simulink model "simpleHelicopter"  (R2024a)
settings: Solver=FixedStepAuto  StartTime=0.0  StopTime=500  FixedStep=fixedStepSize  RelTol=1e-3
model workspace: external: MATLAB File .\turboShaftEngine\Scripts\Initialization\initialization.m (data not in the file)
libraries: fl_lib x4, nesl_utility x3, simulink x2, aerolibatmos2 x1, SignalEditorBlockLib x1
settings Model: DataDictionary=initialization.sldd  EnableAccessToBaseWorkspace=off  Creator=imyrsini  LastModifiedBy=imyrsini
settings OptimizationCC: ZeroExternalMemoryAtStartup=off  ZeroInternalMemoryAtStartup=off
settings RTWCC: TargetLang=C++  GPUComputeCapability=3.5
settings GRTTargetCC: TargetLangStandard=C++11 (ISO)  CodeInterfacePackaging=C++ class
settings SimscapeCC: SimscapeLogSimulationStatistics=on  SimscapeLogToSDI=on  SimscapeLogLimitData=off

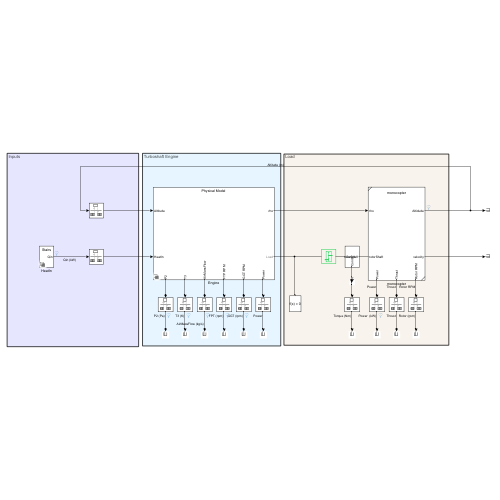
[thumbnail: Simulink's stored preview of the top-level diagram]
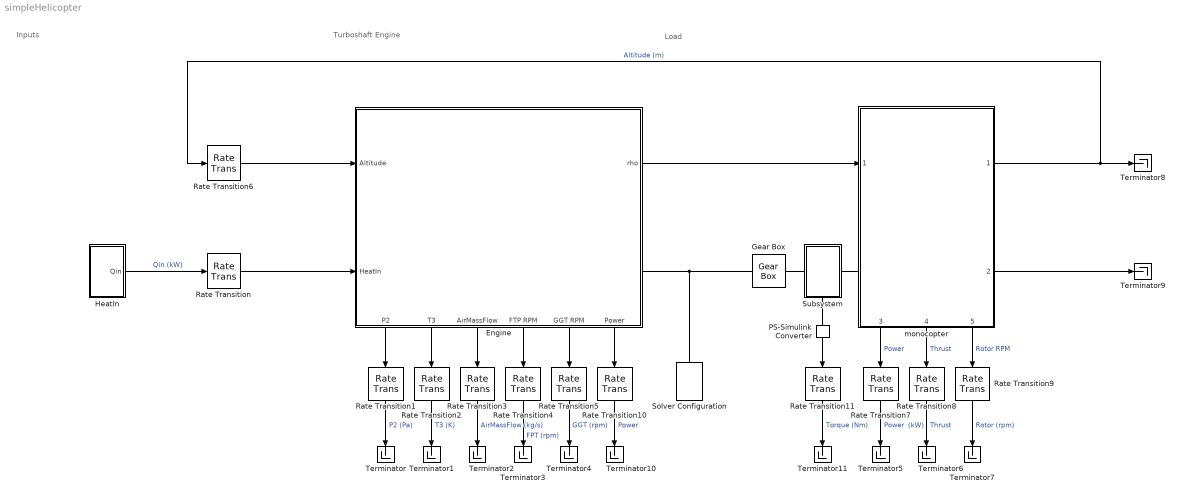
== system simpleHelicopter ==
  note: Load
  note: Turboshaft Engine
  note: Inputs
  Engine : Subsystem  Variant=on  VariantControlMode=label  VariantControl=Subsystem  LabelModeActiveChoice=PhysMod
      settings: PortSchema="{\"entries\":[{\"content\":{\"sides\":[{\"content\":{\"connectorIds\":[\"In1\",\"In2\"]},\"type\":\"ConnectorPlacement.EquallySpacedRectSide\",\"uuid\":\"4b97c1b6-1ef0-4aa6-ad92-ebabb24ed618\"},{\"content\":{\"connectorIds\":[\"Out1\",\"RConn1\"],\"side\":\"RIGHT\"},\"type\":\"ConnectorPlacement.EquallySpacedRectSide\",\"uuid\":\"48732025-ee88-4ad0-bb4a-c439796f910a\"},{\"content\":{\"side\":\"TOP\"},\"type\":\"ConnectorPlacement.EquallySpacedRectSide\",\"uuid\":\"e2101b7b-5c5b-49a6-a3d3-6276ba2fcf7e\"},{\"content\":{\"connectorIds\":[\"Out2\",\"Out3\",\"Out4\",\"Out5\",\"Out6\",\"Out7\"],\"side\":\"BOTTOM\"},\"type\":\"ConnectorPlacement.EquallySpacedRectSide\",\"uuid\":\"1d0ac715-4d03-40bf-a736-541001f37f0a\"}]},\"type\":\"ConnectorPlacement.EquallySpacedConnector\",\"uuid\":\"cc865452-eabe-4ee6-a5dd-432e5e4e603b\"}],\"packageUris\":[\"http://schema.mathworks.com/mf0/Connector/R2020b\"],\"version\":\"1.0\"}"
  Gear Box : fl_lib/Mechanical/Mechanisms/Gear Box  ratio=shaftFTP.GearRatio  t_in_specify=off  t_in_priority=None  t_in=0 N*m  t_in_nominal_specify=off  t_in_nominal_value=1  t_in_nominal_unit=N*m  t_out_specify=off  t_out_priority=None  t_out=0 N*m  t_out_nominal_specify=off  t_out_nominal_value=1  t_out_nominal_unit=N*m
  HeatIn : Subsystem  Variant=on  VariantControlMode=label  VariantControl=Choice  LabelModeActiveChoice=Stairs
  PS-Simulink Converter : nesl_utility/PS-Simulink Converter  PhysicalDomain=network_engine_domain  SubClassName=ps_output  LeftPortType=input  RightPortType=output  PseudoPeriodic=off  Frequencies=[]  VectorFormat=inherit  Unit=inherit  AffineConversion=off
  Rate Transition{,1..11} (12 alike) : RateTransition  Integrity=off
  Solver Configuration : nesl_utility/Solver Configuration  PhysicalDomain=network_engine_domain  SubClassName=solver  LeftPortType=input  RightPortType=generic  Tones=[]  Harmonics=[]  SimulateNoise=off  Profile=off  UseLocalSampling=off  EnableSwitchedLinearOptims=on  FrequencyDomain=off  UseCCode=off  RelTol=0.001  AbsTol=0.001  MinStep=1e-09  ToWorkspace=off  RevertToSquareIcSolve=off  NumHomotopyIterations=100  PhasorMode=off  PhasorModeNumHarmonics=1  ConsistencySolver=NEWTON_XTOL_AFTER_FTOL  IndexReductionMethod=DerivativeReplacement  DoDC=on  ResidualTolerance=1e-09  ConsistencyTolSource=GLOBAL  ConsistencyAbsTol=0.001  ConsistencyRelTol=0.001  ConsistencyTolFactor=0.001  UseLocalSolver=off  LocalSolverChoice=NE_BACKWARD_EULER_ADVANCER  ResolveIndetEquations=on  FunctionEvalNumThread=1  LocalSolverSampleTime=0.001  DoFixedCost=off  MaxNonlinIter=3  MaxModeIter=2  ComputeImpulses=off  ImpulseIterations=2  LinearAlgebra=auto  LinearAlgebraNumThread=0  EquationFormulation=NE_TIME_EF  DelaysMemoryBudget=1024  AutomaticFiltering=on  FilteringTimeConstant=0.001  PartitionStorageMethod=AS_NEEDED  PartitionMemoryBudget=1024  PartitionMethod=ROBUST  MultibodyUseLocalSolver=off  MultibodyLocalSolverChoice=ODE1  MultibodyLocalSolverSampleTime=0.001
  Subsystem : Subsystem
      settings: PortSchema="{\"entries\":[{\"content\":{\"sides\":[{\"content\":{\"connectorIds\":[\"LConn1\"]},\"type\":\"ConnectorPlacement.EquallySpacedRectSide\",\"uuid\":\"cd933ecd-5fe2-4a61-aaa8-d3fcacb54062\"},{\"content\":{\"connectorIds\":[\"RConn1\"],\"side\":\"RIGHT\"},\"type\":\"ConnectorPlacement.EquallySpacedRectSide\",\"uuid\":\"e8204415-45e5-46c1-88c3-e1f0a7c4e852\"},{\"content\":{\"side\":\"TOP\"},\"type\":\"ConnectorPlacement.EquallySpacedRectSide\",\"uuid\":\"484e5189-0a43-4f33-96ac-bd4f306fcf4f\"},{\"content\":{\"connectorIds\":[\"RConn2\"],\"side\":\"BOTTOM\"},\"type\":\"ConnectorPlacement.EquallySpacedRectSide\",\"uuid\":\"524c6b30-eaeb-4c5f-81b0-1e7f5997b042\"}]},\"type\":\"ConnectorPlacement.EquallySpacedConnector\",\"uuid\":\"7bdab1e5-ac38-4f53-a4df-032da561ec46\"}],\"packageUris\":[\"http://schema.mathworks.com/mf0/Connector/R2020b\"],\"version\":\"1.0\"}"
  Terminator{,1..11} (12 alike) : Terminator
  monocopter : Subsystem  ReferencedSubsystem=monocopter
      settings: PortSchema="{\"entries\":[{\"content\":{\"sides\":[{\"content\":{\"connectorIds\":[\"In1\",\"LConn1\"]},\"type\":\"ConnectorPlacement.EquallySpacedRectSide\",\"uuid\":\"2ecbf831-8a46-4c85-bf63-980a752dd5b1\"},{\"content\":{\"connectorIds\":[\"Out1\",\"Out2\"],\"side\":\"RIGHT\"},\"type\":\"ConnectorPlacement.EquallySpacedRectSide\",\"uuid\":\"e1b9456e-2a06-4a0b-bd2d-ca850f525143\"},{\"content\":{\"side\":\"TOP\"},\"type\":\"ConnectorPlacement.EquallySpacedRectSide\",\"uuid\":\"495d5151-b094-4c59-ad95-48151a95ddaf\"},{\"content\":{\"connectorIds\":[\"Out3\",\"Out4\",\"Out5\"],\"side\":\"BOTTOM\"},\"type\":\"ConnectorPlacement.EquallySpacedRectSide\",\"uuid\":\"d711d358-7c2d-4243-addb-9f7f6c9821dd\"}]},\"type\":\"ConnectorPlacement.EquallySpacedConnector\",\"uuid\":\"3949e89b-de6d-4024-bd06-1eddfa87edaa\"}],\"packageUris\":[\"http://schema.mathworks.com/mf0/Connector/R2020b\"],\"version\":\"1.0\"}"
  wires:
  HeatIn/1(Qin) -> Rate Transition/1  "Qin (kW)"
  monocopter/2 -> Terminator9/1
  monocopter/3 -> Rate Transition7/1  "Power"
  monocopter/4 -> Rate Transition8/1  "Thrust"
  monocopter/5 -> Rate Transition9/1  "Rotor RPM"
  monocopter/1 -> Terminator8/1, Rate Transition6/1  "Altitude (m)"
  Rate Transition7/1 -> Terminator5/1  "Power  (kW)"
  Rate Transition8/1 -> Terminator6/1  "Thrust"
  Rate Transition9/1 -> Terminator7/1  "Rotor (rpm)"
  Rate Transition6/1 -> Engine/1(Altitude)
  Rate Transition/1 -> Engine/2(HeatIn)
  Engine/1(rho) -> monocopter/1
  Engine/2(P2) -> Rate Transition1/1
  Engine/3(T3) -> Rate Transition2/1
  Engine/4(AirMassFlow) -> Rate Transition3/1
  Engine/5(FTP RPM) -> Rate Transition4/1
  Engine/6(GGT RPM) -> Rate Transition5/1
  Engine/7(Power) -> Rate Transition10/1
  Rate Transition1/1 -> Terminator/1  "P2 (Pa)"
  Rate Transition2/1 -> Terminator1/1  "T3 (K)"
  Rate Transition3/1 -> Terminator2/1  "AirMassFlow (kg/s)"
  Rate Transition4/1 -> Terminator3/1  "FPT (rpm)"
  Rate Transition5/1 -> Terminator4/1  "GGT (rpm)"
  Rate Transition10/1 -> Terminator10/1  "Power"
  PS-Simulink Converter/1 -> Rate Transition11/1
  Rate Transition11/1 -> Terminator11/1  "Torque (Nm)"
  connections:
  Solver Configuration/RConn1 -- Engine/RConn1 -- Gear Box/LConn1
  Subsystem/RConn1 -- Gear Box/RConn1
  Subsystem/LConn1 -- monocopter/LConn1
  Subsystem/RConn2 -- PS-Simulink Converter/LConn1

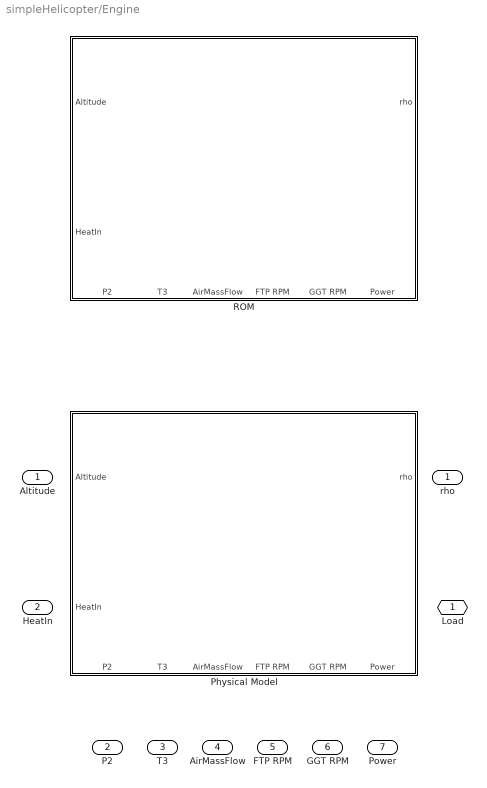
== system simpleHelicopter/Engine ==
  Altitude : Inport
  HeatIn : Inport  Port=2
  Physical Model : Subsystem  VariantControl=PhysMod
      settings: PortSchema="{\"entries\":[{\"content\":{\"sides\":[{\"content\":{\"connectorIds\":[\"In1\",\"In2\"]},\"type\":\"ConnectorPlacement.EquallySpacedRectSide\",\"uuid\":\"4b97c1b6-1ef0-4aa6-ad92-ebabb24ed618\"},{\"content\":{\"connectorIds\":[\"Out1\",\"RConn1\"],\"side\":\"RIGHT\"},\"type\":\"ConnectorPlacement.EquallySpacedRectSide\",\"uuid\":\"48732025-ee88-4ad0-bb4a-c439796f910a\"},{\"content\":{\"side\":\"TOP\"},\"type\":\"ConnectorPlacement.EquallySpacedRectSide\",\"uuid\":\"e2101b7b-5c5b-49a6-a3d3-6276ba2fcf7e\"},{\"content\":{\"connectorIds\":[\"Out2\",\"Out3\",\"Out4\",\"Out5\",\"Out6\",\"Out7\"],\"side\":\"BOTTOM\"},\"type\":\"ConnectorPlacement.EquallySpacedRectSide\",\"uuid\":\"1d0ac715-4d03-40bf-a736-541001f37f0a\"}]},\"type\":\"ConnectorPlacement.EquallySpacedConnector\",\"uuid\":\"cc865452-eabe-4ee6-a5dd-432e5e4e603b\"}],\"packageUris\":[\"http://schema.mathworks.com/mf0/Connector/R2020b\"],\"version\":\"1.0\"}"
  ROM : Subsystem  VariantControl=ROM
      settings: PortSchema="{\"entries\":[{\"content\":{\"sides\":[{\"content\":{\"connectorIds\":[\"In1\",\"In2\"]},\"type\":\"ConnectorPlacement.EquallySpacedRectSide\",\"uuid\":\"4b97c1b6-1ef0-4aa6-ad92-ebabb24ed618\"},{\"content\":{\"connectorIds\":[\"Out1\",\"RConn1\"],\"side\":\"RIGHT\"},\"type\":\"ConnectorPlacement.EquallySpacedRectSide\",\"uuid\":\"48732025-ee88-4ad0-bb4a-c439796f910a\"},{\"content\":{\"side\":\"TOP\"},\"type\":\"ConnectorPlacement.EquallySpacedRectSide\",\"uuid\":\"e2101b7b-5c5b-49a6-a3d3-6276ba2fcf7e\"},{\"content\":{\"connectorIds\":[\"Out2\",\"Out3\",\"Out4\",\"Out5\",\"Out6\",\"Out7\"],\"side\":\"BOTTOM\"},\"type\":\"ConnectorPlacement.EquallySpacedRectSide\",\"uuid\":\"1d0ac715-4d03-40bf-a736-541001f37f0a\"}]},\"type\":\"ConnectorPlacement.EquallySpacedConnector\",\"uuid\":\"cc865452-eabe-4ee6-a5dd-432e5e4e603b\"}],\"packageUris\":[\"http://schema.mathworks.com/mf0/Connector/R2020b\"],\"version\":\"1.0\"}"
  Load : PMIOPort  Side=Right
  rho : Outport
  P2 : Outport  Port=2
  T3 : Outport  Port=3
  AirMassFlow : Outport  Port=4
  FTP RPM : Outport  Port=5
  GGT RPM : Outport  Port=6
  Power : Outport  Port=7

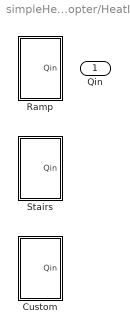
== system simpleHelicopter/HeatIn ==
  Custom : Subsystem  VariantControl=Custom
  Ramp : Subsystem  VariantControl=Ramp
  Stairs : Subsystem  VariantControl=Stairs
  Qin : Outport

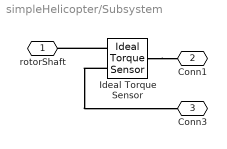
== system simpleHelicopter/Subsystem ==
  Ideal Torque Sensor : fl_lib/Mechanical/Mechanical Sensors/Ideal Torque Sensor
  rotorShaft : PMIOPort  Side=Left
  Conn1 : PMIOPort  Port=2  Side=Right
  Conn3 : PMIOPort  Port=3  Side=Right
  connections:
  Ideal Torque Sensor/RConn2 -- Conn3/RConn1
  Ideal Torque Sensor/LConn1 -- Conn1/RConn1
  Ideal Torque Sensor/RConn1 -- rotorShaft/RConn1

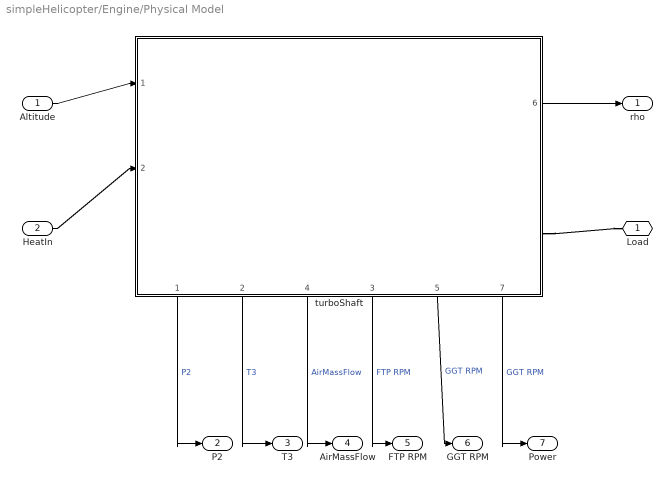
== system simpleHelicopter/Engine/Physical Model ==
  Altitude : Inport
  HeatIn : Inport  Port=2
  turboShaft : Subsystem  ReferencedSubsystem=turboShaft
      settings: PortSchema="{\"entries\":[{\"content\":{\"sides\":[{\"content\":{\"connectorIds\":[\"In1\",\"In2\",\"LConn1\"]},\"type\":\"ConnectorPlacement.EquallySpacedRectSide\",\"uuid\":\"7ef2fcb2-1b0d-44c2-984d-f1d7df0d7e80\"},{\"content\":{\"connectorIds\":[\"Out6\",\"RConn1\"],\"side\":\"RIGHT\"},\"type\":\"ConnectorPlacement.EquallySpacedRectSide\",\"uuid\":\"b2d8a67b-1c6d-4b5e-865c-86345858511b\"},{\"content\":{\"side\":\"TOP\"},\"type\":\"ConnectorPlacement.EquallySpacedRectSide\",\"uuid\":\"4c7a9b07-6c1b-4859-8cda-a5c2cd89c129\"},{\"content\":{\"connectorIds\":[\"Out1\",\"Out2\",\"Out4\",\"Out3\",\"Out5\",\"Out7\"],\"side\":\"BOTTOM\"},\"type\":\"ConnectorPlacement.EquallySpacedRectSide\",\"uuid\":\"794a4e7c-d3e7-4ff8-9cf4-b7022afdc3bd\"}]},\"type\":\"ConnectorPlacement.EquallySpacedConnector\",\"uuid\":\"5f81fd46-9bac-4f96-9ad1-c3a7cd36c01a\"}],\"packageUris\":[\"http://schema.mathworks.com/mf0/Connector/R2020b\"],\"version\":\"1.0\"}"
  Load : PMIOPort  Side=Right
  rho : Outport
  P2 : Outport  Port=2
  T3 : Outport  Port=3
  AirMassFlow : Outport  Port=4
  FTP RPM : Outport  Port=5
  GGT RPM : Outport  Port=6
  Power : Outport  Port=7
  wires:
  turboShaft/2 -> T3/1  "T3"
  turboShaft/5 -> GGT RPM/1  "GGT RPM"
  turboShaft/3 -> FTP RPM/1  "FTP RPM"
  turboShaft/4 -> AirMassFlow/1  "AirMassFlow"
  turboShaft/1 -> P2/1  "P2"
  turboShaft/6 -> rho/1
  HeatIn/1 -> turboShaft/2
  Altitude/1 -> turboShaft/1
  turboShaft/7 -> Power/1  "GGT RPM"
  connections:
  turboShaft/RConn1 -- Load/RConn1

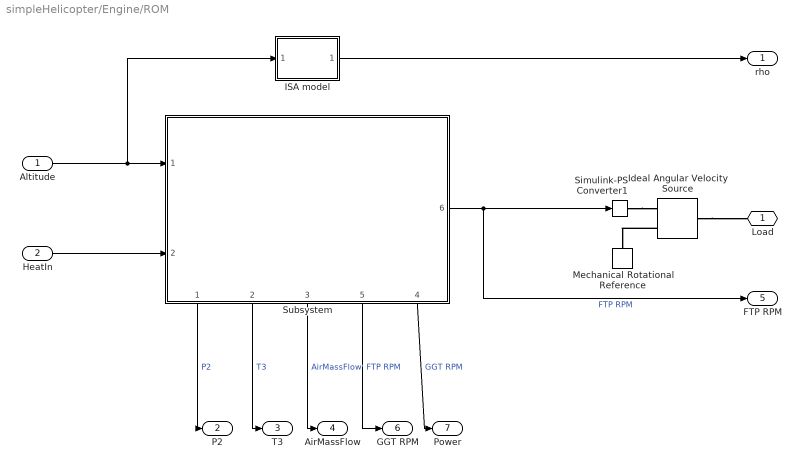
== system simpleHelicopter/Engine/ROM ==
  Altitude : Inport
  HeatIn : Inport  Port=2
  ISA model : Subsystem
  Ideal Angular Velocity Source : fl_lib/Mechanical/Mechanical Sources/Ideal Angular Velocity Source
  Mechanical Rotational Reference : fl_lib/Mechanical/Rotational Elements/Mechanical Rotational Reference
  Simulink-PS Converter1 : nesl_utility/Simulink-PS Converter  PhysicalDomain=network_engine_domain  SubClassName=ps_input  LeftPortType=input  RightPortType=output  PseudoPeriodic=off  Frequencies=[]  NoiseDistribution=none  NoiseParameters=[]  Unit=rpm  AffineConversion=off  FilteringAndDerivatives=filter  SimscapeFilterOrder=2  InputFilterTimeConstant=fixedStepSize  UdotUserProvided=0
  Subsystem : Subsystem  ReferencedSubsystem=lstm_turboShaftEngine
      settings: PortSchema="{\"entries\":[{\"content\":{\"sides\":[{\"content\":{\"connectorIds\":[\"In1\",\"In2\"]},\"type\":\"ConnectorPlacement.EquallySpacedRectSide\",\"uuid\":\"7920ffa2-fa35-490a-8d2a-d5dfbe6c6590\"},{\"content\":{\"connectorIds\":[\"Out6\"],\"side\":\"RIGHT\"},\"type\":\"ConnectorPlacement.EquallySpacedRectSide\",\"uuid\":\"83125dc3-a557-4488-80f1-9e314febf824\"},{\"content\":{\"side\":\"TOP\"},\"type\":\"ConnectorPlacement.EquallySpacedRectSide\",\"uuid\":\"ba262837-84ff-4985-9619-929dd124c29a\"},{\"content\":{\"connectorIds\":[\"Out1\",\"Out2\",\"Out3\",\"Out5\",\"Out4\"],\"side\":\"BOTTOM\"},\"type\":\"ConnectorPlacement.EquallySpacedRectSide\",\"uuid\":\"009c9890-7b19-4ffc-b0a7-3325114fea5d\"}]},\"type\":\"ConnectorPlacement.EquallySpacedConnector\",\"uuid\":\"400dc66e-59e5-4048-8df8-84772b11b1df\"}],\"packageUris\":[\"http://schema.mathworks.com/mf0/Connector/R2020b\"],\"version\":\"1.0\"}"
  Load : PMIOPort  Side=Right
  rho : Outport
  P2 : Outport  Port=2
  T3 : Outport  Port=3
  AirMassFlow : Outport  Port=4
  FTP RPM : Outport  Port=5
  GGT RPM : Outport  Port=6
  Power : Outport  Port=7
  wires:
  Subsystem/4 -> Power/1  "GGT RPM"
  Altitude/1 -> ISA model/1(Height), Subsystem/1
  HeatIn/1 -> Subsystem/2
  Subsystem/1 -> P2/1  "P2"
  Subsystem/3 -> AirMassFlow/1  "AirMassFlow"
  Subsystem/2 -> T3/1  "T3"
  ISA model/1(Outport) -> rho/1
  Subsystem/6 -> Simulink-PS Converter1/1, FTP RPM/1  "FTP RPM"
  Subsystem/5 -> GGT RPM/1  "FTP RPM"
  connections:
  Ideal Angular Velocity Source/RConn2 -- Mechanical Rotational Reference/LConn1
  Ideal Angular Velocity Source/LConn1 -- Load/RConn1
  Simulink-PS Converter1/RConn1 -- Ideal Angular Velocity Source/RConn1

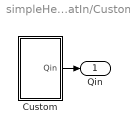
== system simpleHelicopter/HeatIn/Custom ==
  Custom : Subsystem  VariantControl=Custom
  Qin : Outport
  wires:
  Custom/1(Qin) -> Qin/1

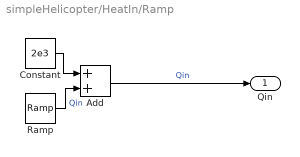
== system simpleHelicopter/HeatIn/Ramp ==
  Add : Sum
  Constant : Constant  Value=2e3
  Ramp : simulink/Sources/Ramp  slope=6  start=rom.init.timeColdStart  InitialOutput=0
  Qin : Outport
  wires:
  Ramp/1 -> Add/2  "Qin"
  Constant/1 -> Add/1
  Add/1 -> Qin/1  "Qin"

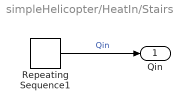
== system simpleHelicopter/HeatIn/Stairs ==
  Repeating Sequence1 : simulink/Sources/Repeating Sequence  rep_seq_t=Qin_time  rep_seq_y=Qin
  Qin : Outport
  wires:
  Repeating Sequence1/1 -> Qin/1  "Qin"

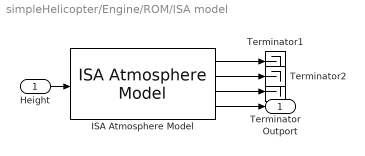
== system simpleHelicopter/Engine/ROM/ISA model ==
  Height : Inport
  ISA Atmosphere Model : aerolibatmos2/ISA Atmosphere Model  useExtended=off  action=Warning  custom=off  viscosityOut=off  g=9.80665  gamma=1.4  R=287.0531  L=0.0065  h_trop=11000  h_strat=20000  rho0=1.225  P0=101325  T0=288.15  h0=0  S=110.4  Tref=273.15  muref=1.716e-5
  Terminator : Terminator
  Terminator1 : Terminator
  Terminator2 : Terminator
  Outport : Outport
  wires:
  ISA Atmosphere Model/4 -> Outport/1
  ISA Atmosphere Model/1 -> Terminator1/1
  Height/1 -> ISA Atmosphere Model/1
  ISA Atmosphere Model/2 -> Terminator2/1
  ISA Atmosphere Model/3 -> Terminator/1

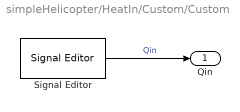
== system simpleHelicopter/HeatIn/Custom/Custom ==
  Signal Editor : SignalEditorBlockLib/Signal Editor  FileName=testScenario.mat  ActiveScenario=Scenario  ActiveSignal=Signal 1  IsBus=off  OutputBusObjectStr=Bus: BusObject  SampleTime=0  ZeroCross=off  OutputAfterFinalValue=Setting to zero  Unit=inherit  PreserveSignalName=on  ApplySigPropsToAllScenarios=on  ApplySigPropsToAllSignals=off
  Qin : Outport
  wires:
  Signal Editor/1 -> Qin/1  "Qin"
